simulink model "sfun_test"  (R2020b)
settings: Solver=VariableStepAuto  StartTime=0.0  StopTime=100  RelTol=1e-3
settings Model: Creator=huang  LastModifiedBy=huang

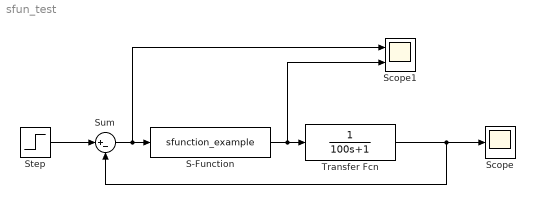
== system sfun_test ==
  S-Function : S-Function  FunctionName=sfunction_example  SFunctionDeploymentMode=off  EnableBusSupport=off
  Scope : Scope
  Scope1 : Scope  NumInputPorts=2
  Step : Step  SampleTime=0
  Sum : Sum  Inputs=|+-
  Transfer Fcn : TransferFcn  Denominator=[100 1]
  wires:
  Step/1 -> Sum/1
  Transfer Fcn/1 -> Sum/2, Scope/1
  Sum/1 -> Scope1/1, S-Function/1
  S-Function/1 -> Scope1/2, Transfer Fcn/1
